simulink model "Hunt_crossley_Ident"  (Simulink 8.0)
settings: Solver=ode3  StartTime=0.0  StopTime=20  FixedStep=0.001  RelTol=1e-3
undefined symbols (not defined in the file): sigbuilder_block
libraries: simulink x2, dspstat3 x1
settings Model: Creator=x  LastModifiedBy=x
settings DebuggingCC: FrameProcessingCompatibilityMsg=error
settings CodeAppCC: CustomSymbolStrType=$N$R$M_T  InternalIdentifier=Shortened
settings GRTTargetCC: CodeReplacementLibrary=None  CPPClassGenCompliant=on

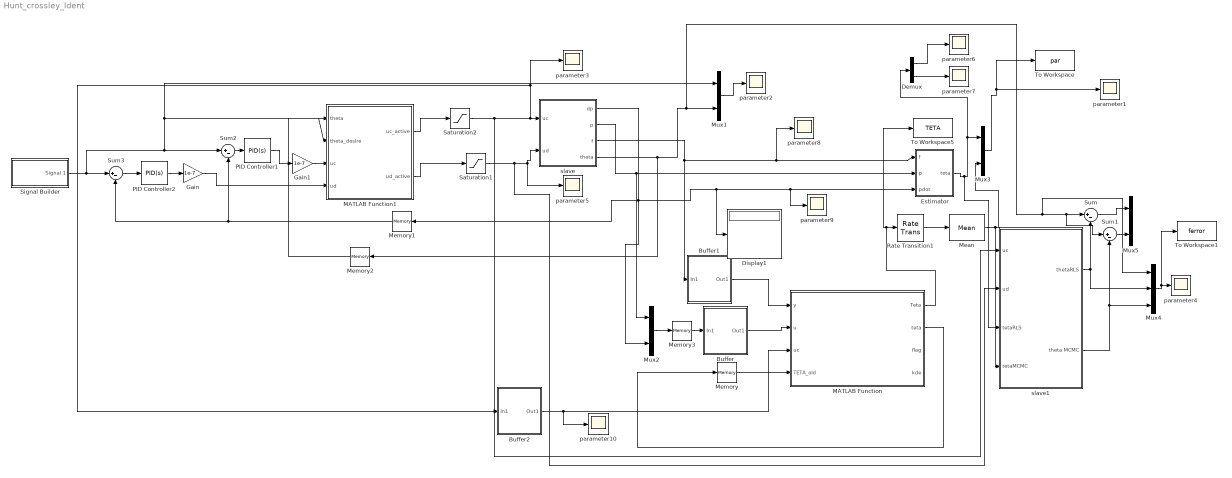
== system Hunt_crossley_Ident ==
  Buffer : Subsystem
  Buffer1 : Subsystem
  Buffer2 : Subsystem
  Demux : Demux  Outputs=2
  Display1 : Display
  Estimator : Subsystem
  Gain : Gain  Gain=1e-7  SampleTime=0.001
  Gain1 : Gain  Gain=1e-7  SampleTime=0.001
  MATLAB Function : MATLAB Function  TreatAsAtomicUnit=on
  MATLAB Function1 : MATLAB Function  TreatAsAtomicUnit=on
  Mean : dspstat3/Mean  run=off  reset_popup=None  InputProcessing=Columns as channels (frame based)  directionMode=Each row  dimension=1  treatSBRowAsCol=on  roiEnable=off  roiType=Rectangles  roiPortion=Entire ROI  roiOutput=Individual statistics for each ROI  roiFlag=off  outputDataTypeStr=Inherit: Same as accumulator  outputLastDataTypeStr=Inherit: Same as accumulator  outputMin=[]  outputMax=[]  roundingMode=Floor  overflowMode=off
  Memory : Memory  X0=[1;1]*1e-5*ones(1,2000)  InheritSampleTime=on
  Memory1 : Memory  InheritSampleTime=on  LinearizeMemory=on
  Memory2 : Memory  InheritSampleTime=on  LinearizeMemory=on
  Memory3 : Memory  X0=[0;0]  InheritSampleTime=on  LinearizeMemory=on
  Mux{1..3,5} (4 alike) : Mux  Inputs=2
  Mux4 : Mux  Inputs=3
  PID Controller1 : simulink/Continuous/PID Controller  Controller=PID  TimeDomain=Continuous-time  SampleTime=0.001  IntegratorMethod=Forward Euler  FilterMethod=Forward Euler  Form=Parallel  P=1  I=0.15  D=0.03  N=100  InitialConditionSource=internal  InitialConditionForIntegrator=0  InitialConditionForFilter=0  ExternalReset=none  LimitOutput=off  UpperSaturationLimit=inf  LowerSaturationLimit=-inf  LinearizeAsGain=on  AntiWindupMode=none  Kb=1  TrackingMode=off  Kt=1  PParamMin=[]  PParamMax=[]  IParamMin=[]  IParamMax=[]  DParamMin=[]  DParamMax=[]  NParamMin=[]  NParamMax=[]  KbParamMin=[]  KbParamMax=[]  KtParamMin=[]  KtParamMax=[]  POutMin=[]  POutMax=[]  IOutMin=[]  IOutMax=[]  DOutMin=[]  DOutMax=[]  NOutMin=[]  NOutMax=[]  KbOutMin=[]  KbOutMax=[]  KtOutMin=[]  KtOutMax=[]  IntegratorOutMin=[]  IntegratorOutMax=[]  FilterOutMin=[]  FilterOutMax=[]  SumOutMin=[]  SumOutMax=[]  SumI1OutMin=[]  SumI1OutMax=[]  SumI2OutMin=[]  SumI2OutMax=[]  SumI3OutMin=[]  SumI3OutMax=[]  SumDOutMin=[]  SumDOutMax=[]  SaturationOutMin=[]  SaturationOutMax=[]  IntegratorContinuousStateAttributes=''  IntegratorStateMustResolveToSignalObject=off  IntegratorRTWStateStorageClass=Auto  FilterContinuousStateAttributes=''  FilterStateMustResolveToSignalObject=off  FilterRTWStateStorageClass=Auto
  PID Controller2 : simulink/Continuous/PID Controller  Controller=PID  TimeDomain=Continuous-time  SampleTime=1  IntegratorMethod=Forward Euler  FilterMethod=Forward Euler  Form=Parallel  P=100  I=30  D=10  N=100  InitialConditionSource=internal  InitialConditionForIntegrator=0  InitialConditionForFilter=0  ExternalReset=none  LimitOutput=off  UpperSaturationLimit=inf  LowerSaturationLimit=-inf  LinearizeAsGain=on  AntiWindupMode=none  Kb=1  TrackingMode=off  Kt=1  PParamMin=[]  PParamMax=[]  IParamMin=[]  IParamMax=[]  DParamMin=[]  DParamMax=[]  NParamMin=[]  NParamMax=[]  KbParamMin=[]  KbParamMax=[]  KtParamMin=[]  KtParamMax=[]  POutMin=[]  POutMax=[]  IOutMin=[]  IOutMax=[]  DOutMin=[]  DOutMax=[]  NOutMin=[]  NOutMax=[]  KbOutMin=[]  KbOutMax=[]  KtOutMin=[]  KtOutMax=[]  IntegratorOutMin=[]  IntegratorOutMax=[]  FilterOutMin=[]  FilterOutMax=[]  SumOutMin=[]  SumOutMax=[]  SumI1OutMin=[]  SumI1OutMax=[]  SumI2OutMin=[]  SumI2OutMax=[]  SumI3OutMin=[]  SumI3OutMax=[]  SumDOutMin=[]  SumDOutMax=[]  SaturationOutMin=[]  SaturationOutMax=[]  IntegratorContinuousStateAttributes=''  IntegratorStateMustResolveToSignalObject=off  IntegratorRTWStateStorageClass=Auto  FilterContinuousStateAttributes=''  FilterStateMustResolveToSignalObject=off  FilterRTWStateStorageClass=Auto
  Rate Transition1 : RateTransition  X0=ones(2,1501)*1e-7  OutPortSampleTime=0.001
  Saturation1 : Saturate  UpperLimit=1  LowerLimit=0  SampleTime=0.001
  Saturation2 : Saturate  UpperLimit=1  LowerLimit=0  SampleTime=0.001
  Signal Builder : Subsystem  Tag=STV Subsys  LoadFcn=sigbuilder_block('load');  StartFcn=sigbuilder_block('start');  StopFcn=sigbuilder_block('stop');  ClipboardFcn=sigbuilder_block('clipboard');  mask(Sigbuilder block){}
      mask help: Simulink:masks:SigbuilderBlock_MD
      mask init:
      | if ~strcmp(get_param(bdroot(gcbh),'SimulationStatus'),'stopped') tuvar = sigbuilder_block('maskInit'); end
      settings: CopyFcn=sigbuilder_block('copy');  DeleteFcn=sigbuilder_block('delete');  ModelCloseFcn=sigbuilder_block('modelClose');  PreSaveFcn=sigbuilder_block('preSave');  PauseFcn=sigbuilder_block('pause');  ContinueFcn=sigbuilder_block('continue');  NameChangeFcn=sigbuilder_block('namechange');  OpenFcn=sigbuilder_block('open',[160.138 11.1724 549.931 396 ]);  CloseFcn=sigbuilder_block('close');
      mask Display: plot(0, 0, 100, 100,[2, 2, 32, 32, 2], [68, 8, 8, 68, 68],[32, 2], [38, 38], [32, 19, 2],[53, 60, 44], [32, 17, 17, 2],[16, 16, 31, 31]);txt = getActiveGroup(gcbh);text(2, 100, txt,'verticalAlignment', 'top');
  Sum{,1..3} (4 alike) : Sum  Inputs=|+-
  To Workspace : ToWorkspace  VariableName=par  SampleTime=-1
  To Workspace1 : ToWorkspace  VariableName=ferror  SampleTime=-1
  To Workspace5 : ToWorkspace  VariableName=TETA  SampleTime=-1
  parameter{1..10} (10 alike) : Scope
      parameter10 settings: TimeRange=20  YMin=0  YMax=1.5  SaveName=ScopeData8
      parameter2 settings: TimeRange=20  YMin=0  YMax=1.5
      parameter3 settings: SaveName=ScopeData2
      parameter5 settings: TimeRange=20  YMin=-80000000000  YMax=70000000000  SaveName=ScopeData3
      parameter6 settings: TimeRange=20  YMin=3.4e-13  YMax=3.75e-13  SaveName=ScopeData4
      parameter7 settings: TimeRange=10  YMin=-2e-15  YMax=4e-15  SaveName=ScopeData6
      parameter8 settings: TimeRange=20  SaveName=ScopeData5
      parameter9 settings: TimeRange=20  YMin=0  YMax=1.5  SaveName=ScopeData7
  slave : Subsystem
  slave1 : Subsystem
  wires:
  Mux2/1 -> Memory3/1
  MATLAB Function/2(teta) -> Memory/1
  Buffer/1(Out1) -> MATLAB Function/2(u)
  Rate Transition1/1 -> Mean/1
  Memory/1 -> MATLAB Function/4(TETA_old)
  Mux3/1 -> To Workspace/1, parameter1/1
  Estimator/1(teta) -> slave1/3(tetaRLS), Mux3/1, Demux/1
  slave/2(p) -> Estimator/2(p), Mux2/1
  Mux4/1 -> To Workspace1/1, parameter4/1
  MATLAB Function/1(Teta) -> To Workspace5/1, Rate Transition1/1
  Mean/1 -> slave1/4(tetaMCMC), Mux3/2
  slave1/1("thetaRLS ") -> Mux4/2, Sum/2
  Sum/1 -> Mux5/1
  slave1/2(theta MCMC) -> Sum1/2, Mux4/3
  Sum1/1 -> Mux5/2
  Signal Builder/1(Signal 1) -> MATLAB Function1/2(theta_desire), Mux1/1, Sum2/1, Sum3/1
  Sum2/1 -> PID Controller1/1
  Sum3/1 -> PID Controller2/1
  PID Controller2/1 -> Gain/1
  PID Controller1/1 -> Gain1/1
  slave/3(f) -> Buffer1/1(In1), parameter8/1, Estimator/1(f)
  Mux1/1 -> parameter2/1
  slave/4("theta ") -> Memory2/1, Mux4/1, Sum1/1, Sum/1, Mux1/2
  Memory2/1 -> MATLAB Function1/1(theta)
  Memory1/1 -> Sum2/2, Sum3/2
  Demux/1 -> parameter6/1
  Demux/2 -> parameter7/1
  Memory3/1 -> Buffer/1(In1)
  Buffer1/1(Out1) -> MATLAB Function/1(y)
  Buffer2/1(Out1) -> parameter10/1, MATLAB Function/3(uc)
  Saturation2/1 -> Buffer2/1(In1), parameter3/1, slave/1(uc), slave1/1(uc)
  Saturation1/1 -> slave1/2(ud), slave/2(ud), parameter5/1
  MATLAB Function1/1(uc_active) -> Saturation2/1
  MATLAB Function1/2(ud_active) -> Saturation1/1
  Gain1/1 -> MATLAB Function1/3(uc)
  Gain/1 -> MATLAB Function1/4(ud)
  slave/1(dp) -> Memory1/1, Mux2/2, Display1/1, parameter9/1, Estimator/3(pdot)

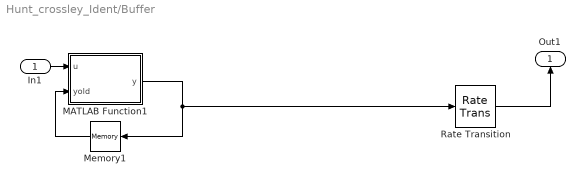
== system Hunt_crossley_Ident/Buffer ==
  In1 : Inport
  MATLAB Function1 : MATLAB Function  TreatAsAtomicUnit=on
  Memory1 : Memory  X0=zeros(100,2)  LinearizeMemory=on
  Rate Transition : RateTransition  X0=zeros(100,2)  OutPortSampleTime=0.1
  Out1 : Outport
  wires:
  Rate Transition/1 -> Out1/1
  Memory1/1 -> MATLAB Function1/2(yold)
  In1/1 -> MATLAB Function1/1(u)
  MATLAB Function1/1(y) -> Rate Transition/1, Memory1/1

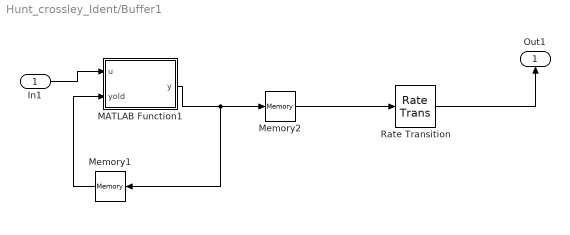
== system Hunt_crossley_Ident/Buffer1 ==
  In1 : Inport
  MATLAB Function1 : MATLAB Function  TreatAsAtomicUnit=on
  Memory1 : Memory  X0=zeros(100,1)  LinearizeMemory=on
  Memory2 : Memory  X0=zeros(100,1)  LinearizeMemory=on
  Rate Transition : RateTransition  X0=zeros(100,1)  OutPortSampleTime=0.1
  Out1 : Outport
  wires:
  Memory1/1 -> MATLAB Function1/2(yold)
  Memory2/1 -> Rate Transition/1
  MATLAB Function1/1(y) -> Memory2/1, Memory1/1
  In1/1 -> MATLAB Function1/1(u)
  Rate Transition/1 -> Out1/1

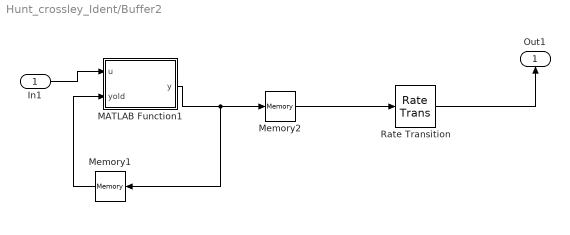
== system Hunt_crossley_Ident/Buffer2 ==
  In1 : Inport
  MATLAB Function1 : MATLAB Function  TreatAsAtomicUnit=on
  Memory1 : Memory  X0=zeros(100,1)  LinearizeMemory=on
  Memory2 : Memory  X0=zeros(100,1)  LinearizeMemory=on
  Rate Transition : RateTransition  X0=zeros(100,1)  OutPortSampleTime=0.1
  Out1 : Outport
  wires:
  Rate Transition/1 -> Out1/1
  In1/1 -> MATLAB Function1/1(u)
  MATLAB Function1/1(y) -> Memory1/1, Memory2/1
  Memory2/1 -> Rate Transition/1
  Memory1/1 -> MATLAB Function1/2(yold)

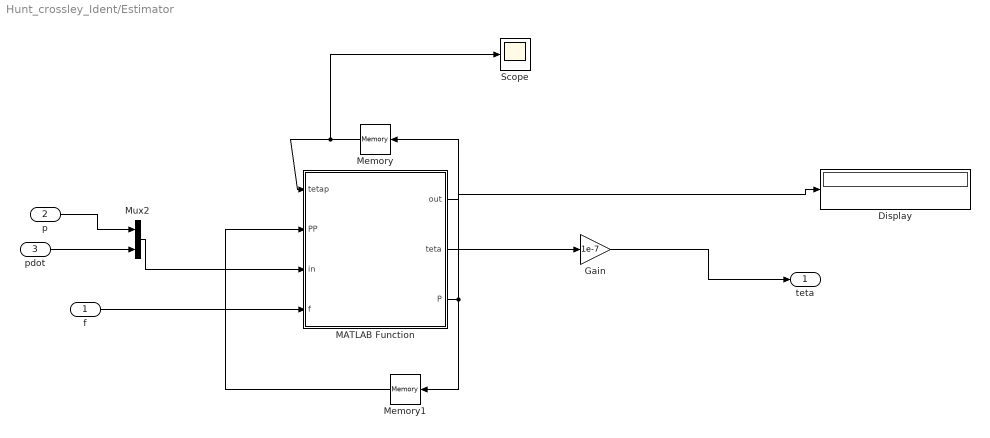
== system Hunt_crossley_Ident/Estimator ==
  f : Inport
  p : Inport  Port=2
  pdot : Inport  Port=3
  Display : Display
  Gain : Gain  Gain=1e-7
  MATLAB Function : MATLAB Function  TreatAsAtomicUnit=on
  Memory : Memory  X0=[-2.14e-4,6.12e-9]*0
  Memory1 : Memory  X0=1e5*[1 0;0 1]
  Mux2 : Mux  Inputs=2
  Scope : Scope
  teta : Outport
  wires:
  f/1 -> MATLAB Function/4(f)
  MATLAB Function/1(out) -> Memory/1
  Memory1/1 -> MATLAB Function/2(PP)
  Mux2/1 -> MATLAB Function/3(in)
  Memory/1 -> Scope/1, MATLAB Function/1(tetap)
  pdot/1 -> Mux2/2
  p/1 -> Mux2/1
  MATLAB Function/3(P) -> Memory1/1, Display/1
  MATLAB Function/2(teta) -> Gain/1
  Gain/1 -> teta/1

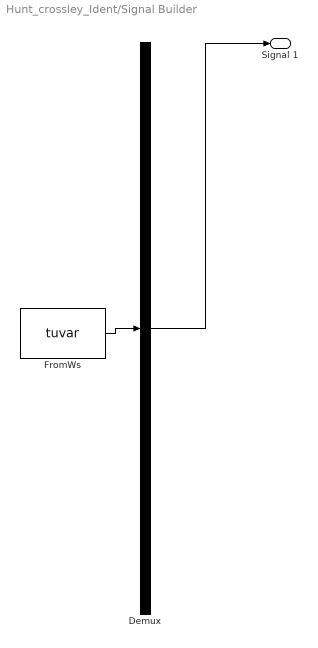
== system Hunt_crossley_Ident/Signal Builder ==
  Demux : Demux  Tag=STV Demux  Outputs=1
  FromWs : FromWorkspace  Tag=STV FromWs  VariableName=tuvar  SampleTime=0  SigBuilderData=DataTag1  VnvData=DataTag2
      SigBuilderData=|
      | common.afterFinalStr = 'Extrapolate'
      | common.sampleTime = 0
      | dataSet.timeRange = [0 20]
      | dataSet.name = 'Group 1'
      | sbobj.Groups.Name = 'Group 1'
      | sbobj.Groups.Signals.Name = 'Signal 1'
      | sbobj.Groups.Signals.XData = [0 5 5 14 14 20]
      | sbobj.Groups.Signals.YData = [0.8 0.8 0.195 0.195 1.4 1.4]
      | sbobj.Groups.TimeRange = [0 20]
  Signal 1 : Outport  Tag=STV Outport
  wires:
  Demux/1 -> Signal 1/1
  FromWs/1 -> Demux/1

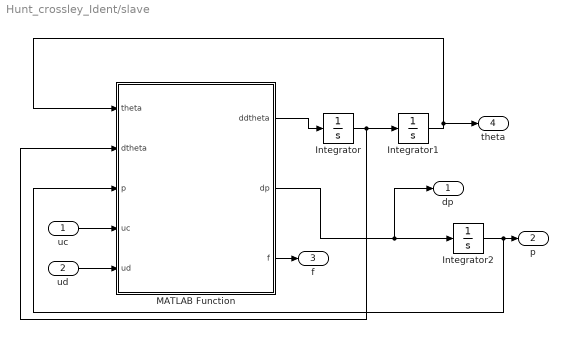
== system Hunt_crossley_Ident/slave ==
  uc : Inport
  ud : Inport  Port=2
  Integrator : Integrator
  Integrator1 : Integrator
  Integrator2 : Integrator  InitialCondition=101.325e3
  MATLAB Function : MATLAB Function  TreatAsAtomicUnit=on
  dp : Outport
  p : Outport  Port=2
  f : Outport  Port=3
  "theta " : Outport  Port=4
  wires:
  uc/1 -> MATLAB Function/4(uc)
  ud/1 -> MATLAB Function/5(ud)
  MATLAB Function/1(ddtheta) -> Integrator/1
  Integrator/1 -> MATLAB Function/2(dtheta), Integrator1/1
  MATLAB Function/2(dp) -> dp/1, Integrator2/1
  Integrator2/1 -> MATLAB Function/3(p), p/1
  MATLAB Function/3(f) -> f/1
  Integrator1/1 -> "theta "/1, MATLAB Function/1(theta)

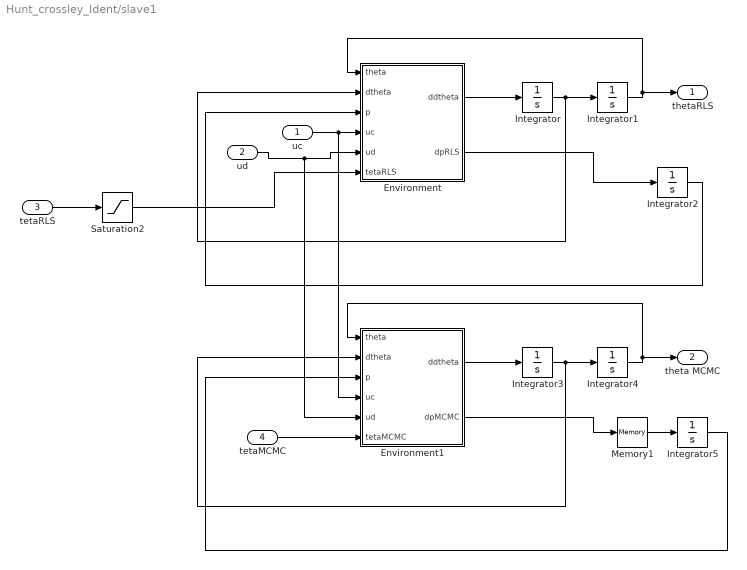
== system Hunt_crossley_Ident/slave1 ==
  uc : Inport
  ud : Inport  Port=2
  tetaRLS : Inport  Port=3
  tetaMCMC : Inport  Port=4
  Environment : MATLAB Function  TreatAsAtomicUnit=on
  Environment1 : MATLAB Function  TreatAsAtomicUnit=on
  Integrator{,1,3..4} (4 alike) : Integrator
  Integrator2 : Integrator  InitialCondition=101.325e3
  Integrator5 : Integrator  InitialCondition=101.325e3
  Memory1 : Memory  InheritSampleTime=on  LinearizeMemory=on
  Saturation2 : Saturate  UpperLimit=1  LowerLimit=0  SampleTime=0.001
  "thetaRLS " : Outport
  theta MCMC : Outport  Port=2
  wires:
  Environment/1(ddtheta) -> Integrator/1
  Integrator/1 -> Environment/2(dtheta), Integrator1/1
  Environment/2(dpRLS) -> Integrator2/1
  Integrator2/1 -> Environment/3(p)
  Integrator1/1 -> Environment/1(theta), "thetaRLS "/1
  tetaRLS/1 -> Saturation2/1
  uc/1 -> Environment1/4(uc), Environment/4(uc)
  ud/1 -> Environment1/5(ud), Environment/5(ud)
  Environment1/1(ddtheta) -> Integrator3/1
  Integrator3/1 -> Environment1/2(dtheta), Integrator4/1
  Environment1/2(dpMCMC) -> Memory1/1
  Integrator5/1 -> Environment1/3(p)
  Integrator4/1 -> Environment1/1(theta), theta MCMC/1
  tetaMCMC/1 -> Environment1/6(tetaMCMC)
  Memory1/1 -> Integrator5/1
  Saturation2/1 -> Environment/6(tetaRLS)

== matlab function slave/MATLAB Function ==
  data: theta input double; dtheta input double; p input double; uc input double; ddtheta output double; ud input double; dp output double; f output double
function [ddtheta,dp,f] = fcn(theta,dtheta,p,uc,ud)
%parameter

t1 = 1408.50;
t2 = 132.28;
t3 = 3319.40;
t4 = -2.14e-4;
t5 = 6.12e-9;
t6 = -9.76e-5;
t7 = -1.9e-9;
patm = 101.325e3;
ps = 800e3;


ddtheta = t1*(p-patm)-t2*dtheta-t3*theta;
if uc>0
    f = uc*sign(ps-p)*sqrt(abs(ps-p));
    dp =(t4+t5*p)\f;
else
    f = ud*sign(p-patm)*sqrt(abs(p-patm));
    dp =(t6+t7*p)\f;
end

== matlab function MATLAB Function ==
  data: Teta output double; y input double; u input double; uc input double; TETA_old input double; teta output double; flag output double; kde output double
function [Teta,teta,flag,kde]  = online_enhanced_mcmc(y,u ,uc ,TETA_old)
coder.extrinsic('ksdensity');
coder.extrinsic('unifrnd');
kde_y=zeros(1,100);
kde_x=zeros(1,100);
kde=zeros(2,100);
n=100;
lambda=0.95;
SampNum=2000;
nac=0;
count = 0;
ParNum = 2;
sigma2_RW = 1e-7;
sigma2 = 3e-3;   
% preallcoation for speed
epsi=zeros(ParNum, 1);
ye1=0;
flag=0; %noninformative prior
inint_ths=0.01;
init_low=-0.01;
init_high=0.01;
SampMin=1000;
AccMin=0.9;
npdf=1/sqrt(2*pi*sigma2^2);

ye1_candid = 0;

%%%%%%%%%%%%%%%%%%%%%%%%%%%% special cases (flag=2)%%%%%%%%%%%%%%%%%%%%%%%%%%%%%%%%%%%
% no environment
for i2 = 1:n
    if (abs(u(i2,2))<1e-5 )
        count=count+1;
    end
end
% start up
if count>0.1*n
    teta=TETA_old;
    flag=2;
else
    
%%%%%%%%%%%%%%%%%%%%%%%%%%%% Normal cases (flag!=2)%%%%%%%%%%%%%%%%%%%%%%%%%%%%%%%%%%%
  %--------------------- Initializing -----------------------------------
dummy=0;
teta=[TETA_old(:,2:end), (mean(TETA_old(:,floor(SampNum/2):end)'))'];
for i2 = 1:n
    %ye1(i2) = u(i2,:) * teta(:,end) ;
    dumm=u(i2,2)*(teta(1,end)+u(i2,1)*teta(2,end));
    if dumm <0
        dummy=-inf;
        break;
    end
    ye1 = log10(abs(u(i2,2)))+log10(abs(teta(1,end)+u(i2,1)*teta(2,end))) ;
    dummy=log10(npdf*exp(-(exp(-lambda*(n-i2)))*(y(i2) - 10^ye1)^2/sigma2^2))+dummy;
    %dummy = log10(normpdf(y(i2) - ye1(i2), 0, sigma2)) + dummy;
end




if 10^dummy>inint_ths
    prob_teta = dummy;
%%%%%%%%%%%%%%%%%%%% informative prior (flag=1)%%%%%%%%%%%%%%%%%%%%%%%%%%    
    sigma2_RW=0.01*sigma2_RW;
 for  k = 1:SampNum
      
        %-------------------- Introducing Candidate ---------------------------
%                          epsi(:,k) = teta(:,k) + normrnd(0,sqrt(sigma2_RW),[size(teta,1),1]);
          epsi= teta(:,ceil(rand*ParNum))+sqrt(sigma2_RW)*randn([size(teta,1),1]); 
                            

        %-------------------- Evaluating Acceptance ---------------------------

        % Prior Knowledg
        if (( epsi(1)>0 ) ||( epsi(1)<-1e-3 ) || (epsi(2)> 1e-7) ||(epsi(2)< -1e-7))
            prob_epsi = -inf;
        else

            ye1_candid = 0;
            dummy = 0; % Computing Probability of Epsilon Parameter
            for i2 = 1:n
                % ---- Computing candidate probability accordance to noise distribution ----

%                 ye1_candid(i2) =  u(i2,:) * epsi(:);
                 dumm= u(i2,2)*(epsi(1)+u(i2,1)*epsi(2));
                 
                 if dumm<0
                     dummy=-inf;
                     break;
                 end
                ye1_candid =log10(abs(u(i2,2)))+log10(abs(epsi(1)+u(i2,1)*epsi(2))) ;
                
                

                %dummy = log10(normpdf(y(i2) - ye1_candid(i2), 0,sigma2)) + dummy;
                dummy=log10(npdf*exp(-(exp(-lambda*(n-i2)))*(y(i2) - 10^ye1_candid)^2/sigma2^2))+dummy;

            end

            prob_epsi = dummy;

        end
        alpha = min(1,10^(prob_epsi-prob_teta));
        z = rand(1,1);
        
            if (z < alpha)
                teta = [teta(:,2:end), epsi];
                prob_teta = prob_epsi;
                nac=nac+1;
            else
                teta = [teta(:,2:end), teta(:,end)];
            end
            
            if (k>SampMin && nac <k*AccMin)
                break;
            end
            if (k==floor(0.75*SampMin) && nac <0.5*k*AccMin)
                sigma2_RW=0.1*sigma2_RW;
            end
            if (k==0.5*SampMin && nac <0.5*k*AccMin)
                sigma2_RW=0.1*sigma2_RW;
            end
      
 end
   
   flag=1; 
end


%%%%%%%%%%%%%%%%%%%% non informative prior (flag=0)%%%%%%%%%%%%%%%%%%%%%%%%%%
if flag==0
dummy = -inf;
%while (isinf(dummy))
 while (10^dummy<10^22)
     if mean(uc)>0 
         teta(1,1) = unifrnd(-1e-3,-1e-4,1);
         teta(2,1) = unifrnd(0,1e-7,1);
     else
         teta(1,1) = unifrnd(-1e-4,-1e-5,1);
         teta(2,1) = unifrnd(-1e-7,0,1);
     end
    count = 0;
    dummy = 0; % Computing Probability of Previous Sample Parameter
            
   % ye1 = 0; 
            
    for i2 = 1:n
       
%            ye1(i2) = u(i2,:) * teta(:,1);
            dumm = u(i2,2)*(teta(1,1)+u(i2,1)*teta(2,1));
            if dumm<0
                count = count +1;
            end
            if count>0.03*n
                dummy=-inf;
                break;
            end
           ye1 = log10(abs(u(i2,2)))+log10(abs(teta(1,1)+u(i2,1)*teta(2,1)));
                    % -------- Computing first step of MCMC accordance to noise type ------
           %dummy = log10(normpdf(y(i2) - ye1(i2), 0, sigma2)) + dummy ;
           dummy=log10(npdf*exp(-(exp(-lambda*(n-i2)))*(y(i2) - 10^ye1)^2/sigma2^2))+dummy;

           if isinf(dummy)
                 break;
           end

    end

    prob_teta = dummy; 
%     count = count + 1
end

for  k = 1:(SampNum-1)
    
    prob_teta = dummy;
      
        %-------------------- Introducing Candidate ---------------------------
                     
               epsi = teta(:,k) +sqrt(sigma2_RW)*randn([size(teta,1),1]);
                      
        %-------------------- Evaluating Acceptance ---------------------------
          % Prior Knowledg
        if (( epsi(1)>0 ) ||( epsi(1)<-1e-3 ) || (epsi(2)> 1e-7) ||(epsi(2)< -1e-7)) 
            prob_epsi = -inf;
        else

            ye1_candid = 0;
            dummy = 0; % Computing Probability of Epsilon Parameter
            for i2 = 1:n
                % ---- Computing candidate probability accordance to noise distribution ----

%                 ye1_candid(i2) =  u(i2,:) * epsi(:);
                
                dumm= u(i2,2)*(epsi(1)+u(i2,1)*epsi(2));
                 
                 if dumm<0
                     dummy=-inf;
                     break;
                 end
                ye1_candid =log10(abs(u(i2,2)))+log10(abs(epsi(1)+u(i2,1)*epsi(2))) ;

                %dummy = log10(normpdf(y(i2) - ye1_candid(i2), 0,sigma2)) + dummy;
                dummy=log10(npdf*exp(-(exp(-lambda*(n-i2)))*(y(i2) - 10^ye1_candid)^2/sigma2^2))+dummy;

            end

            prob_epsi = dummy;

        end

        alpha = min(1,10^(prob_epsi-prob_teta));
        z = rand(1,1);
        
            if (z < alpha)
                teta(:,k+1) = epsi;
                prob_teta = prob_epsi;
                nac=nac+1;
            else
                teta(:,k+1) = teta(:,k);
            end
            
           % if (k>2*SampMin && nac<0.5*k*AccMin)
           %     break;
           % end
            if (k==floor(1.5*SampMin) && nac <0.5*k*AccMin)
                sigma2_RW=0.5*sigma2_RW;
            end
            if (k==2*SampMin && nac <0.8*k*AccMin)
                sigma2_RW=0.5*sigma2_RW;
            end
end
end
    
%nac=nac/k;
end


[kde_x,kde_y]=ksdensity(teta(1,500:end));
kde=[kde_x ;kde_y];
%plot(kde_y ,kde_x);
[kde_x,kde_y]=ksdensity(teta(2,500:end));
%%figure(2);
%%plot(kde_y ,kde_x);
%[kde_x,kde_y]=ksdensity(teta(3,500:end));
%figure(3);
%plot(kde_y ,kde_x);
Teta=teta(:,500:end);
end

== matlab function Estimator/MATLAB Function ==
  data: out output double; tetap input double; PP input double; in input double; f input double; teta output double; P output double
function [out, teta, P]= fcn(tetap,   PP,   in,   f)
%parameter
landa=1;
% if ( f<0)
%    out=[1;1];
%    teta=[0;0];
%    P=10^3*eye(2,2);
% else

phi=[in(2);in(1)*in(2)];
%scalling
phi = phi*1e-7;

L=PP*phi/(landa+phi'*PP*phi);
P=1/landa*(PP-L*phi'*PP);
out=tetap+L*(f-phi'*tetap);
teta=[out(1); out(2)];


if (P(1,1)>1e5)
    P(1,1)=1e5;
end
if (P(2,2)>1e5)
     P(2,2)=1e5;
end
end

== matlab function Buffer/MATLAB Function1 ==
  data: u input double; y output double; yold input double
function y = fcn(u,yold)
%#codegen

y = [yold(2:100,:);u'];

== matlab function MATLAB Function1 ==
  data: uc_active output double; theta input double; theta_desire input double; uc input double; ud input double; ud_active output double
function [uc_active,ud_active] = fcn(theta,theta_desire,uc,ud)
%#codegen

if theta_desire>theta
    uc_active = uc(1);
    ud_active = ud*0;
else
    uc_active = uc*0;
    ud_active = ud(1);
end
end

== matlab function Buffer1/MATLAB Function1 ==
  data: u input double; y output double; yold input double
function y = fcn(u,yold)
%#codegen

y = [yold(2:100);u];

== matlab function Buffer2/MATLAB Function1 ==
  data: u input double; y output double; yold input double
function y = fcn(u,yold)
%#codegen

y = [yold(2:100);u];

== matlab function slave1/Environment1 ==
  data: ddtheta output double; theta input double; dtheta input double; p input double; uc input double; ud input double; tetaMCMC input double; dpMCMC output double
function [ddtheta, dpMCMC]= ENV( theta, dtheta, p,uc,ud ,tetaMCMC)
%   Parameter
p1=tetaMCMC(1);p2=tetaMCMC(2); 
t1 = 1408.50;
t2 = 132.28;
t3 = 3319.40;
patm = 101.325e3;
ps = 800e3;

ddtheta = t1*(p-patm)-t2*dtheta-t3*theta;
if uc>0
    f = uc*sign(ps-p)*sqrt(abs(ps-p));
else
    f = ud*sign(p-patm)*sqrt(abs(p-patm));
end

dpMCMC =(p1+p2*p)\f;
end

== matlab function slave1/Environment ==
  data: ddtheta output double; theta input double; dtheta input double; p input double; uc input double; ud input double; tetaRLS input double; dpRLS output double
function [ddtheta, dpRLS]= ENV( theta, dtheta, p,uc,ud ,tetaRLS)
%   Parameter
p1=tetaRLS(1);p2=tetaRLS(2); 
t1 = 1408.50;
t2 = 132.28;
t3 = 3319.40;
patm = 101.325e3;
ps = 800e3;

ddtheta = t1*(p-patm)-t2*dtheta-t3*theta;
if uc>0
    f = uc*sign(ps-p)*sqrt(abs(ps-p));
else
    f = ud*sign(p-patm)*sqrt(abs(p-patm));
end

dpRLS =(p1+p2*p)\f;
end
